simulink model "ROBOT_OK"  (R2021a)
settings: Solver=FixedStepAuto  StartTime=0.0  StopTime=inf  FixedStep=0.001  RelTol=1e-3
model workspace: external: MATLAB File E:\2024\TINH_TOAN_ROBOT_6_DOF\ROBOT_OK_DataFile.m (data not in the file)
values from neighbouring files (symbols this model uses):
  X = Toado(:,1)    [QuydaoK.m]
  Y = Toado(:,2)    [QuydaoK.m]
  Z = Toado(:,3)    [QuydaoK.m]
undefined symbols (not defined in the file or in its folder): smiData
libraries: sm_lib x38, nesl_utility x30, sharedutil x16, sharedtransform x12, dspmtrx3 x12, simulink_extras x8, pid_lib x6, simulink x3
(part 1 of 6)
settings Model: EnablePacing=on  Creator=NGAI-LAPTOP  LastModifiedBy=NGAI-LAPTOP

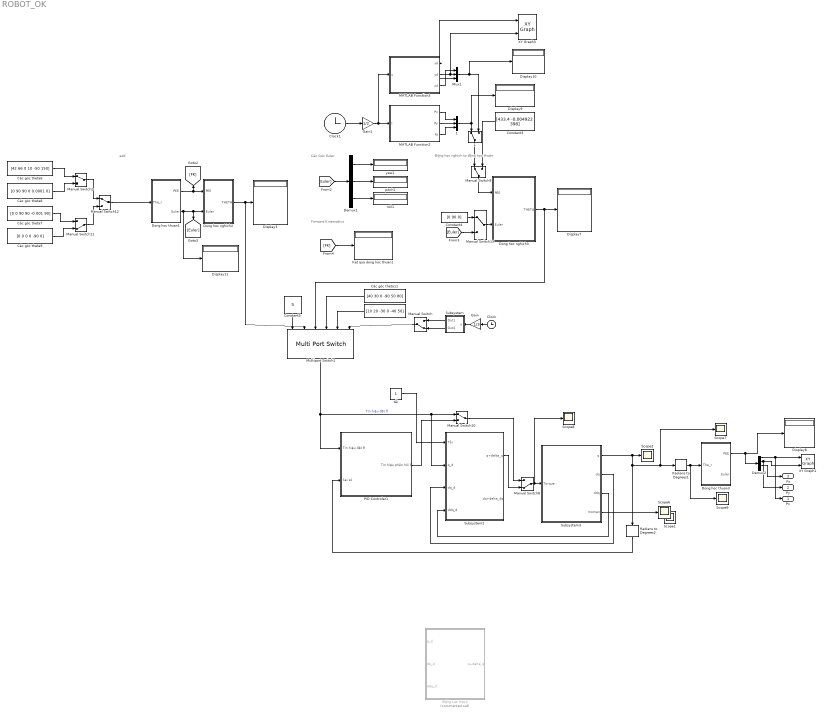
== system ROBOT_OK ==
  note: Động học nghịch to động học thuận
  note: Các Góc Euler
  note: add
  note: Forward Kinematics
  "   " : Constant  Value=[10 20 -30 0 -40 50]
  "   1" : Mux  Inputs=3
  " 1" : ManualSwitch
  Clock : Clock
  Clock1 : Clock
  Constant3 : Constant  Value=[433.4 -0.004922 398]
  Constant4 : Constant  Value=[0 90 0]
  Constant5 : Constant  Value=5
  Các góc theta11 : Constant  Value=[40 30 0 -90 50 80]
  Các góc theta6 : Constant  Value=[42 66 0 10 -50 150]
  Các góc theta7 : Constant  Value=[0 0 90 90 -0.001 90]
  Các góc theta8 : Constant  Value=[0 90 90 0 0.0001 0]
  Các góc theta9 : Constant  Value=[0 0 0 0 -90 0]
  Demux1 : Demux  Outputs=3
  Demux2 : Demux
  Display{3,7..11} (6 alike) : Display
  Dong hoc nghich2 : Subsystem
  Dong hoc nghich3 : Subsystem
  Dong hoc thuan1 : Subsystem
  Dong hoc thuan3 : Subsystem
  Gain : Gain  Gain=1/3
  Gain1 : Gain  Gain=1/2
  Ket qua dong hoc thuan1 : Display
  MATLAB Function2 : MATLAB Function  TreatAsAtomicUnit=on
  MATLAB Function3 : MATLAB Function  TreatAsAtomicUnit=on
  Manual Switch : ManualSwitch  CurrentSetting=0
  Manual Switch{2,9..10,12..13} (5 alike) : ManualSwitch
  Manual Switch11 : ManualSwitch  CurrentSetting=0
  Manual Switch8 : ManualSwitch  CurrentSetting=0
  Multiport Switch1 : MultiPortSwitch  Inputs=5
  Mux1 : Mux  Inputs=3
  PID Controler1 : Subsystem
  Radians to Degrees1 : simulink_extras/Transformations/Radians to Degrees
  Radians to Degrees2 : simulink_extras/Transformations/Radians to Degrees
  Scope{1..2,6..9} (6 alike) : Scope
  Subsystem : Subsystem
  Subsystem2 : Subsystem
  Subsystem3 : Subsystem
  XY Graph1 : simulink/Sinks/XY Graph  xmin=-1000  xmax=1000  ymin=-1000  ymax=1000  st=-1
  XY Graph3 : simulink/Sinks/XY Graph  xmin=-1  xmax=1  ymin=-1  ymax=1  st=-1
  pitch1 : Display
  roll1 : Display
  tải : Constant
  yaw1 : Display
  Động Lực Học2 : Subsystem  Commented=on
  Px : Outport
  Py : Outport  Port=2
  Pz : Outport  Port=3
  wires:
  MATLAB Function3/1(xd) -> Mux1/3, XY Graph3/1
  Các góc theta7/1 -> Manual Switch11/1
  Demux2/3 -> Pz/1
  Demux2/1 -> XY Graph1/1, Px/1
  Manual Switch9/1 -> Dong hoc nghich3/1(PEE)
  Manual Switch8/1 -> Subsystem3/1(Torque), Scope8/1
  Demux1/1 -> yaw1/1
  Manual Switch2/1 -> Manual Switch12/1
  Manual Switch13/1 -> Dong hoc nghich3/2(Euler)
  Subsystem3/4(momen) -> Scope6/1
  Dong hoc thuan3/1(PEE) -> Demux2/1, Display8/1
  [Euler] -> Demux1/1
  Các góc theta6/1 -> Manual Switch2/1
  PID Controler1/1(Tín hiệu phản hồi θ) -> Manual Switch10/2
  Multiport Switch1/1 -> Subsystem2/2(q_d), Manual Switch10/1, PID Controler1/1(Tín hiệu đặt θ)  "Tín hiệu đặt θ"
  Constant4/1 -> Manual Switch13/1
  Constant5/1 -> Multiport Switch1/1
  Radians to Degrees2/1 -> PID Controler1/2(Sai số)
  [FK] -> Ket qua dong hoc thuan1/1
  Manual Switch11/1 -> Manual Switch12/2
  Manual Switch10/1 -> Manual Switch8/1
  Các góc theta11/1 -> Multiport Switch1/4
  Các góc theta9/1 -> Manual Switch11/2
  "   "/1 -> Multiport Switch1/5
  Subsystem2/1(q+delta_q) -> Manual Switch8/2
  [Euler] -> Manual Switch13/2
  " 1"/1 -> Manual Switch9/1
  Subsystem3/2(dq) -> Subsystem2/3(dq_d)
  MATLAB Function3/3(zd) -> Mux1/1
  MATLAB Function3/2(yd) -> Mux1/2, XY Graph3/2
  MATLAB Function2/2(Py) -> "   1"/2
  Subsystem3/3(ddq) -> Subsystem2/4(ddq_d)
  Dong hoc thuan1/1(PEE) -> Dong hoc nghich2/1(PEE), [FK]
  "   1"/1 -> Display9/1, " 1"/1
  Mux1/1 -> " 1"/2, Display10/1
  MATLAB Function2/1(Px) -> "   1"/1
  Demux1/2 -> pitch1/1
  Demux1/3 -> roll1/1
  Gain1/1 -> MATLAB Function3/1(u), MATLAB Function2/1(t)
  MATLAB Function2/3(Pz) -> "   1"/3
  Constant3/1 -> Manual Switch9/2
  Subsystem3/1(q) -> Scope2/1, Radians to Degrees2/1, Radians to Degrees1/1, Scope7/1
  Manual Switch12/1 -> Dong hoc thuan1/1(The_r)
  Dong hoc thuan1/2(Euler) -> Dong hoc nghich2/2(Euler), [Euler], Display11/1
  Các góc theta8/1 -> Manual Switch2/2
  Dong hoc nghich3/1(THETA) -> Multiport Switch1/3, Display7/1
  Dong hoc nghich2/1(THETA) -> Multiport Switch1/2, Display3/1
  Clock1/1 -> Gain1/1
  Radians to Degrees1/1 -> Dong hoc thuan3/1(The_r), Scope9/1
  Demux2/2 -> XY Graph1/2, Py/1
  Subsystem/1(Out1) -> Manual Switch/1
  Subsystem/2(Out2) -> Manual Switch/2
  Manual Switch/1 -> Multiport Switch1/6
  Gain/1 -> Subsystem/1(u)
  Clock/1 -> Gain/1
  tải/1 -> Subsystem2/1(Tải)

== system ROBOT_OK/Dong hoc nghich2 ==
  PEE : Inport
  Euler : Inport  Port=2
  DONG HOC NGHICH : MATLAB Function  TreatAsAtomicUnit=on
  Demux : Demux  Outputs=3
  Display : Display
  Display1 : Display
  Mux : Mux  Inputs=6
  THETA : Outport
  wires:
  Demux/3 -> DONG HOC NGHICH/4(roll)
  Demux/1 -> DONG HOC NGHICH/2(yaw)
  Demux/2 -> DONG HOC NGHICH/3(pitch)
  DONG HOC NGHICH/3(the3) -> Mux/3
  DONG HOC NGHICH/4(the4) -> Mux/4
  DONG HOC NGHICH/2(the2) -> Mux/2
  DONG HOC NGHICH/6(the6) -> Mux/6
  DONG HOC NGHICH/5(the5) -> Mux/5
  PEE/1 -> Display/1, DONG HOC NGHICH/1(P_EE)
  Euler/1 -> Display1/1, Demux/1
  DONG HOC NGHICH/1(the1) -> Mux/1
  Mux/1 -> THETA/1

== system ROBOT_OK/Dong hoc nghich3 ==
  PEE : Inport
  Euler : Inport  Port=2
  DONG HOC NGHICH : MATLAB Function  TreatAsAtomicUnit=on
  Demux : Demux  Outputs=3
  Display : Display
  Display1 : Display
  Mux : Mux  Inputs=6
  THETA : Outport
  wires:
  Demux/3 -> DONG HOC NGHICH/4(roll)
  Demux/1 -> DONG HOC NGHICH/2(yaw)
  Demux/2 -> DONG HOC NGHICH/3(pitch)
  DONG HOC NGHICH/3(the3) -> Mux/3
  DONG HOC NGHICH/4(the4) -> Mux/4
  DONG HOC NGHICH/2(the2) -> Mux/2
  DONG HOC NGHICH/6(the6) -> Mux/6
  DONG HOC NGHICH/5(the5) -> Mux/5
  PEE/1 -> Display/1, DONG HOC NGHICH/1(P_EE)
  Euler/1 -> Display1/1, Demux/1
  DONG HOC NGHICH/1(the1) -> Mux/1
  Mux/1 -> THETA/1

== system ROBOT_OK/Dong hoc thuan1 ==
  The_r : Inport
  DONG HOC THUAN : MATLAB Function  TreatAsAtomicUnit=on
  Demux : Demux  Outputs=6
  Mux : Mux  Inputs=3
  PEE : Outport  VectorParamsAs1DForOutWhenUnconnected=off
  Euler : Outport  Port=2  VectorParamsAs1DForOutWhenUnconnected=off
  wires:
  Demux/5 -> DONG HOC THUAN/5(the5)
  Demux/1 -> DONG HOC THUAN/1(the1)
  Demux/4 -> DONG HOC THUAN/4(the4)
  DONG HOC THUAN/4(roll) -> Mux/3
  Demux/2 -> DONG HOC THUAN/2(the2)
  Demux/3 -> DONG HOC THUAN/3(the3)
  Demux/6 -> DONG HOC THUAN/6(the6)
  The_r/1 -> Demux/1
  DONG HOC THUAN/2(yaw) -> Mux/1
  DONG HOC THUAN/3(pitch) -> Mux/2
  Mux/1 -> Euler/1
  DONG HOC THUAN/1(P_EE) -> PEE/1

== system ROBOT_OK/Dong hoc thuan3 ==
  The_r : Inport
  DONG HOC THUAN : MATLAB Function  TreatAsAtomicUnit=on
  Demux : Demux  Outputs=6
  Mux : Mux  Inputs=3
  PEE : Outport  VectorParamsAs1DForOutWhenUnconnected=off
  Euler : Outport  Port=2  VectorParamsAs1DForOutWhenUnconnected=off
  wires:
  Demux/5 -> DONG HOC THUAN/5(the5)
  Demux/1 -> DONG HOC THUAN/1(the1)
  Demux/4 -> DONG HOC THUAN/4(the4)
  DONG HOC THUAN/4(roll) -> Mux/3
  Demux/2 -> DONG HOC THUAN/2(the2)
  Demux/3 -> DONG HOC THUAN/3(the3)
  Demux/6 -> DONG HOC THUAN/6(the6)
  The_r/1 -> Demux/1
  DONG HOC THUAN/2(yaw) -> Mux/1
  DONG HOC THUAN/3(pitch) -> Mux/2
  Mux/1 -> Euler/1
  DONG HOC THUAN/1(P_EE) -> PEE/1

== system ROBOT_OK/PID Controler1 ==
  Tín hiệu đặt θ : Inport
  Sai số : Inport  Port=2
  Demux1 : Demux  Outputs=6
  Mux : Mux  Inputs=6
  PID Controller1 : pid_lib/PID Controller  Controller=PID  Form=Parallel  TimeDomain=Continuous-time  UseExternalTs=off  SampleTime=-1  IntegratorMethod=Forward Euler  FilterMethod=Forward Euler  ControllerParametersSource=internal  P=0  I=9.99999999999999  D=0  UseFilter=on  N=100  TunerSelectOption=Transfer Function Based (PID Tuner App)  InitialConditionSource=internal  InitialConditionForIntegrator=0  InitialConditionForFilter=0  DifferentiatorICPrevScaledInput=0  ExternalReset=none  TrackingMode=off  Kt=1  LimitOutput=off  SatLimitsSource=internal  UpperSaturationLimit=inf  LowerSaturationLimit=-inf  LinearizeAsGain=on  AntiWindupMode=none  Kb=1  POutMin=[]  POutMax=[]  IOutMin=[]  IOutMax=[]  DOutMin=[]  DOutMax=[]  NOutMin=[]  NOutMax=[]  SumOutMin=[]  SumOutMax=[]  SaturationOutMin=[]  SaturationOutMax=[]  PParamMin=[]  PParamMax=[]  IParamMin=[]  IParamMax=[]  DParamMin=[]  DParamMax=[]  NParamMin=[]  NParamMax=[]  KbParamMin=[]  KbParamMax=[]  KtParamMin=[]  KtParamMax=[]  KbOutMin=[]  KbOutMax=[]  KtOutMin=[]  KtOutMax=[]  IntegratorOutMin=[]  IntegratorOutMax=[]  FilterOutMin=[]  FilterOutMax=[]  SumI1OutMin=[]  SumI1OutMax=[]  SumI2OutMin=[]  SumI2OutMax=[]  SumI3OutMin=[]  SumI3OutMax=[]  SumI4OutMin=[]  SumI4OutMax=[]  SumDOutMin=[]  SumDOutMax=[]  DifferentiatorOutMin=[]  DifferentiatorOutMax=[]  FilterDiffOutCoefMin=[]  FilterDiffOutCoefMax=[]  ReciprocalOutMin=[]  ReciprocalOutMax=[]  SumDenOutMin=[]  SumDenOutMax=[]  SumNumOutMin=[]  SumNumOutMax=[]  DivideOutMin=[]  DivideOutMax=[]  UdiffTsProdOutMin=[]  UdiffTsProdOutMax=[]  NTsProdOutMin=[]  NTsProdOutMax=[]  UintegralTsProdOutMin=[]  UintegralTsProdOutMax=[]  UngainTsProdOutMin=[]  UngainTsProdOutMax=[]  IntegratorContinuousStateAttributes=''  IntegratorStateMustResolveToSignalObject=off  IntegratorRTWStateStorageClass=Auto  FilterContinuousStateAttributes=''  FilterStateMustResolveToSignalObject=off  FilterRTWStateStorageClass=Auto  ParallelPVariant=InternalParameters  IdealPVariant=Disabled  IVariant=InternalParameters  DVariant=InternalParameters  IntegratorVariant=Continuous  SatVariant=Disabled  AWVariant=Passthrough  PCopyVariant=Disabled  TRVariant=Disabled  FdbkBlocksVariant=Forward  IdealPFdbkVariant=Disabled  SatFdbkVariant=Disabled  DerivativeFilterVariant=ContFilter  NVariant=InternalParameters  NCopyVariant=Disabled  FilterICVariant=InternalICsFilter  IntegratorICVariant=InternalICs  ExternalResetVariant=Disabled  TRSumVariant=Passthrough  SumFdbkVariant=Disabled  SumVariant=Sum_PID  TsampFilterVariant=InternalTs  TsampNgainVariant=Passthrough  TsampIntegralVariant=Passthrough  ExternalSaturationOutDataTypeStr=Inherit: Same as second input
  PID Controller2 : pid_lib/PID Controller  Controller=PID  Form=Parallel  TimeDomain=Continuous-time  UseExternalTs=off  SampleTime=-1  IntegratorMethod=Forward Euler  FilterMethod=Forward Euler  ControllerParametersSource=internal  P=0  I=10  D=0  UseFilter=on  N=100  TunerSelectOption=Transfer Function Based (PID Tuner App)  InitialConditionSource=internal  InitialConditionForIntegrator=0  InitialConditionForFilter=0  DifferentiatorICPrevScaledInput=0  ExternalReset=none  TrackingMode=off  Kt=1  LimitOutput=off  SatLimitsSource=internal  UpperSaturationLimit=inf  LowerSaturationLimit=-inf  LinearizeAsGain=on  AntiWindupMode=none  Kb=1  POutMin=[]  POutMax=[]  IOutMin=[]  IOutMax=[]  DOutMin=[]  DOutMax=[]  NOutMin=[]  NOutMax=[]  SumOutMin=[]  SumOutMax=[]  SaturationOutMin=[]  SaturationOutMax=[]  PParamMin=[]  PParamMax=[]  IParamMin=[]  IParamMax=[]  DParamMin=[]  DParamMax=[]  NParamMin=[]  NParamMax=[]  KbParamMin=[]  KbParamMax=[]  KtParamMin=[]  KtParamMax=[]  KbOutMin=[]  KbOutMax=[]  KtOutMin=[]  KtOutMax=[]  IntegratorOutMin=[]  IntegratorOutMax=[]  FilterOutMin=[]  FilterOutMax=[]  SumI1OutMin=[]  SumI1OutMax=[]  SumI2OutMin=[]  SumI2OutMax=[]  SumI3OutMin=[]  SumI3OutMax=[]  SumI4OutMin=[]  SumI4OutMax=[]  SumDOutMin=[]  SumDOutMax=[]  DifferentiatorOutMin=[]  DifferentiatorOutMax=[]  FilterDiffOutCoefMin=[]  FilterDiffOutCoefMax=[]  ReciprocalOutMin=[]  ReciprocalOutMax=[]  SumDenOutMin=[]  SumDenOutMax=[]  SumNumOutMin=[]  SumNumOutMax=[]  DivideOutMin=[]  DivideOutMax=[]  UdiffTsProdOutMin=[]  UdiffTsProdOutMax=[]  NTsProdOutMin=[]  NTsProdOutMax=[]  UintegralTsProdOutMin=[]  UintegralTsProdOutMax=[]  UngainTsProdOutMin=[]  UngainTsProdOutMax=[]  IntegratorContinuousStateAttributes=''  IntegratorStateMustResolveToSignalObject=off  IntegratorRTWStateStorageClass=Auto  FilterContinuousStateAttributes=''  FilterStateMustResolveToSignalObject=off  FilterRTWStateStorageClass=Auto  ParallelPVariant=InternalParameters  IdealPVariant=Disabled  IVariant=InternalParameters  DVariant=InternalParameters  IntegratorVariant=Continuous  SatVariant=Disabled  AWVariant=Passthrough  PCopyVariant=Disabled  TRVariant=Disabled  FdbkBlocksVariant=Forward  IdealPFdbkVariant=Disabled  SatFdbkVariant=Disabled  DerivativeFilterVariant=ContFilter  NVariant=InternalParameters  NCopyVariant=Disabled  FilterICVariant=InternalICsFilter  IntegratorICVariant=InternalICs  ExternalResetVariant=Disabled  TRSumVariant=Passthrough  SumFdbkVariant=Disabled  SumVariant=Sum_PID  TsampFilterVariant=InternalTs  TsampNgainVariant=Passthrough  TsampIntegralVariant=Passthrough  ExternalSaturationOutDataTypeStr=Inherit: Same as second input
  PID Controller3 : pid_lib/PID Controller  Controller=PID  Form=Parallel  TimeDomain=Continuous-time  UseExternalTs=off  SampleTime=-1  IntegratorMethod=Forward Euler  FilterMethod=Forward Euler  ControllerParametersSource=internal  P=0  I=10  D=0  UseFilter=on  N=944.848611425355  TunerSelectOption=Transfer Function Based (PID Tuner App)  InitialConditionSource=internal  InitialConditionForIntegrator=0  InitialConditionForFilter=0  DifferentiatorICPrevScaledInput=0  ExternalReset=none  TrackingMode=off  Kt=1  LimitOutput=off  SatLimitsSource=internal  UpperSaturationLimit=inf  LowerSaturationLimit=-inf  LinearizeAsGain=on  AntiWindupMode=none  Kb=1  POutMin=[]  POutMax=[]  IOutMin=[]  IOutMax=[]  DOutMin=[]  DOutMax=[]  NOutMin=[]  NOutMax=[]  SumOutMin=[]  SumOutMax=[]  SaturationOutMin=[]  SaturationOutMax=[]  PParamMin=[]  PParamMax=[]  IParamMin=[]  IParamMax=[]  DParamMin=[]  DParamMax=[]  NParamMin=[]  NParamMax=[]  KbParamMin=[]  KbParamMax=[]  KtParamMin=[]  KtParamMax=[]  KbOutMin=[]  KbOutMax=[]  KtOutMin=[]  KtOutMax=[]  IntegratorOutMin=[]  IntegratorOutMax=[]  FilterOutMin=[]  FilterOutMax=[]  SumI1OutMin=[]  SumI1OutMax=[]  SumI2OutMin=[]  SumI2OutMax=[]  SumI3OutMin=[]  SumI3OutMax=[]  SumI4OutMin=[]  SumI4OutMax=[]  SumDOutMin=[]  SumDOutMax=[]  DifferentiatorOutMin=[]  DifferentiatorOutMax=[]  FilterDiffOutCoefMin=[]  FilterDiffOutCoefMax=[]  ReciprocalOutMin=[]  ReciprocalOutMax=[]  SumDenOutMin=[]  SumDenOutMax=[]  SumNumOutMin=[]  SumNumOutMax=[]  DivideOutMin=[]  DivideOutMax=[]  UdiffTsProdOutMin=[]  UdiffTsProdOutMax=[]  NTsProdOutMin=[]  NTsProdOutMax=[]  UintegralTsProdOutMin=[]  UintegralTsProdOutMax=[]  UngainTsProdOutMin=[]  UngainTsProdOutMax=[]  IntegratorContinuousStateAttributes=''  IntegratorStateMustResolveToSignalObject=off  IntegratorRTWStateStorageClass=Auto  FilterContinuousStateAttributes=''  FilterStateMustResolveToSignalObject=off  FilterRTWStateStorageClass=Auto  ParallelPVariant=InternalParameters  IdealPVariant=Disabled  IVariant=InternalParameters  DVariant=InternalParameters  IntegratorVariant=Continuous  SatVariant=Disabled  AWVariant=Passthrough  PCopyVariant=Disabled  TRVariant=Disabled  FdbkBlocksVariant=Forward  IdealPFdbkVariant=Disabled  SatFdbkVariant=Disabled  DerivativeFilterVariant=ContFilter  NVariant=InternalParameters  NCopyVariant=Disabled  FilterICVariant=InternalICsFilter  IntegratorICVariant=InternalICs  ExternalResetVariant=Disabled  TRSumVariant=Passthrough  SumFdbkVariant=Disabled  SumVariant=Sum_PID  TsampFilterVariant=InternalTs  TsampNgainVariant=Passthrough  TsampIntegralVariant=Passthrough  ExternalSaturationOutDataTypeStr=Inherit: Same as second input
  PID Controller4 : pid_lib/PID Controller  Controller=PID  Form=Parallel  TimeDomain=Continuous-time  UseExternalTs=off  SampleTime=-1  IntegratorMethod=Forward Euler  FilterMethod=Forward Euler  ControllerParametersSource=internal  P=0  I=10  D=0  UseFilter=on  N=208.357752355368  TunerSelectOption=Transfer Function Based (PID Tuner App)  InitialConditionSource=internal  InitialConditionForIntegrator=0  InitialConditionForFilter=0  DifferentiatorICPrevScaledInput=0  ExternalReset=none  TrackingMode=off  Kt=1  LimitOutput=off  SatLimitsSource=internal  UpperSaturationLimit=inf  LowerSaturationLimit=-inf  LinearizeAsGain=on  AntiWindupMode=none  Kb=1  POutMin=[]  POutMax=[]  IOutMin=[]  IOutMax=[]  DOutMin=[]  DOutMax=[]  NOutMin=[]  NOutMax=[]  SumOutMin=[]  SumOutMax=[]  SaturationOutMin=[]  SaturationOutMax=[]  PParamMin=[]  PParamMax=[]  IParamMin=[]  IParamMax=[]  DParamMin=[]  DParamMax=[]  NParamMin=[]  NParamMax=[]  KbParamMin=[]  KbParamMax=[]  KtParamMin=[]  KtParamMax=[]  KbOutMin=[]  KbOutMax=[]  KtOutMin=[]  KtOutMax=[]  IntegratorOutMin=[]  IntegratorOutMax=[]  FilterOutMin=[]  FilterOutMax=[]  SumI1OutMin=[]  SumI1OutMax=[]  SumI2OutMin=[]  SumI2OutMax=[]  SumI3OutMin=[]  SumI3OutMax=[]  SumI4OutMin=[]  SumI4OutMax=[]  SumDOutMin=[]  SumDOutMax=[]  DifferentiatorOutMin=[]  DifferentiatorOutMax=[]  FilterDiffOutCoefMin=[]  FilterDiffOutCoefMax=[]  ReciprocalOutMin=[]  ReciprocalOutMax=[]  SumDenOutMin=[]  SumDenOutMax=[]  SumNumOutMin=[]  SumNumOutMax=[]  DivideOutMin=[]  DivideOutMax=[]  UdiffTsProdOutMin=[]  UdiffTsProdOutMax=[]  NTsProdOutMin=[]  NTsProdOutMax=[]  UintegralTsProdOutMin=[]  UintegralTsProdOutMax=[]  UngainTsProdOutMin=[]  UngainTsProdOutMax=[]  IntegratorContinuousStateAttributes=''  IntegratorStateMustResolveToSignalObject=off  IntegratorRTWStateStorageClass=Auto  FilterContinuousStateAttributes=''  FilterStateMustResolveToSignalObject=off  FilterRTWStateStorageClass=Auto  ParallelPVariant=InternalParameters  IdealPVariant=Disabled  IVariant=InternalParameters  DVariant=InternalParameters  IntegratorVariant=Continuous  SatVariant=Disabled  AWVariant=Passthrough  PCopyVariant=Disabled  TRVariant=Disabled  FdbkBlocksVariant=Forward  IdealPFdbkVariant=Disabled  SatFdbkVariant=Disabled  DerivativeFilterVariant=ContFilter  NVariant=InternalParameters  NCopyVariant=Disabled  FilterICVariant=InternalICsFilter  IntegratorICVariant=InternalICs  ExternalResetVariant=Disabled  TRSumVariant=Passthrough  SumFdbkVariant=Disabled  SumVariant=Sum_PID  TsampFilterVariant=InternalTs  TsampNgainVariant=Passthrough  TsampIntegralVariant=Passthrough  ExternalSaturationOutDataTypeStr=Inherit: Same as second input
  PID Controller5 : pid_lib/PID Controller  Controller=PID  Form=Parallel  TimeDomain=Continuous-time  UseExternalTs=off  SampleTime=-1  IntegratorMethod=Forward Euler  FilterMethod=Forward Euler  ControllerParametersSource=internal  P=0  I=10  D=0  UseFilter=on  N=100  TunerSelectOption=Transfer Function Based (PID Tuner App)  InitialConditionSource=internal  InitialConditionForIntegrator=0  InitialConditionForFilter=0  DifferentiatorICPrevScaledInput=0  ExternalReset=none  TrackingMode=off  Kt=1  LimitOutput=off  SatLimitsSource=internal  UpperSaturationLimit=inf  LowerSaturationLimit=-inf  LinearizeAsGain=on  AntiWindupMode=none  Kb=1  POutMin=[]  POutMax=[]  IOutMin=[]  IOutMax=[]  DOutMin=[]  DOutMax=[]  NOutMin=[]  NOutMax=[]  SumOutMin=[]  SumOutMax=[]  SaturationOutMin=[]  SaturationOutMax=[]  PParamMin=[]  PParamMax=[]  IParamMin=[]  IParamMax=[]  DParamMin=[]  DParamMax=[]  NParamMin=[]  NParamMax=[]  KbParamMin=[]  KbParamMax=[]  KtParamMin=[]  KtParamMax=[]  KbOutMin=[]  KbOutMax=[]  KtOutMin=[]  KtOutMax=[]  IntegratorOutMin=[]  IntegratorOutMax=[]  FilterOutMin=[]  FilterOutMax=[]  SumI1OutMin=[]  SumI1OutMax=[]  SumI2OutMin=[]  SumI2OutMax=[]  SumI3OutMin=[]  SumI3OutMax=[]  SumI4OutMin=[]  SumI4OutMax=[]  SumDOutMin=[]  SumDOutMax=[]  DifferentiatorOutMin=[]  DifferentiatorOutMax=[]  FilterDiffOutCoefMin=[]  FilterDiffOutCoefMax=[]  ReciprocalOutMin=[]  ReciprocalOutMax=[]  SumDenOutMin=[]  SumDenOutMax=[]  SumNumOutMin=[]  SumNumOutMax=[]  DivideOutMin=[]  DivideOutMax=[]  UdiffTsProdOutMin=[]  UdiffTsProdOutMax=[]  NTsProdOutMin=[]  NTsProdOutMax=[]  UintegralTsProdOutMin=[]  UintegralTsProdOutMax=[]  UngainTsProdOutMin=[]  UngainTsProdOutMax=[]  IntegratorContinuousStateAttributes=''  IntegratorStateMustResolveToSignalObject=off  IntegratorRTWStateStorageClass=Auto  FilterContinuousStateAttributes=''  FilterStateMustResolveToSignalObject=off  FilterRTWStateStorageClass=Auto  ParallelPVariant=InternalParameters  IdealPVariant=Disabled  IVariant=InternalParameters  DVariant=InternalParameters  IntegratorVariant=Continuous  SatVariant=Disabled  AWVariant=Passthrough  PCopyVariant=Disabled  TRVariant=Disabled  FdbkBlocksVariant=Forward  IdealPFdbkVariant=Disabled  SatFdbkVariant=Disabled  DerivativeFilterVariant=ContFilter  NVariant=InternalParameters  NCopyVariant=Disabled  FilterICVariant=InternalICsFilter  IntegratorICVariant=InternalICs  ExternalResetVariant=Disabled  TRSumVariant=Passthrough  SumFdbkVariant=Disabled  SumVariant=Sum_PID  TsampFilterVariant=InternalTs  TsampNgainVariant=Passthrough  TsampIntegralVariant=Passthrough  ExternalSaturationOutDataTypeStr=Inherit: Same as second input
  PID Controller6 : pid_lib/PID Controller  Controller=PID  Form=Parallel  TimeDomain=Continuous-time  UseExternalTs=off  SampleTime=-1  IntegratorMethod=Forward Euler  FilterMethod=Forward Euler  ControllerParametersSource=internal  P=0  I=10  D=0  UseFilter=on  N=100  TunerSelectOption=Transfer Function Based (PID Tuner App)  InitialConditionSource=internal  InitialConditionForIntegrator=0  InitialConditionForFilter=0  DifferentiatorICPrevScaledInput=0  ExternalReset=none  TrackingMode=off  Kt=1  LimitOutput=off  SatLimitsSource=internal  UpperSaturationLimit=inf  LowerSaturationLimit=-inf  LinearizeAsGain=on  AntiWindupMode=none  Kb=1  POutMin=[]  POutMax=[]  IOutMin=[]  IOutMax=[]  DOutMin=[]  DOutMax=[]  NOutMin=[]  NOutMax=[]  SumOutMin=[]  SumOutMax=[]  SaturationOutMin=[]  SaturationOutMax=[]  PParamMin=[]  PParamMax=[]  IParamMin=[]  IParamMax=[]  DParamMin=[]  DParamMax=[]  NParamMin=[]  NParamMax=[]  KbParamMin=[]  KbParamMax=[]  KtParamMin=[]  KtParamMax=[]  KbOutMin=[]  KbOutMax=[]  KtOutMin=[]  KtOutMax=[]  IntegratorOutMin=[]  IntegratorOutMax=[]  FilterOutMin=[]  FilterOutMax=[]  SumI1OutMin=[]  SumI1OutMax=[]  SumI2OutMin=[]  SumI2OutMax=[]  SumI3OutMin=[]  SumI3OutMax=[]  SumI4OutMin=[]  SumI4OutMax=[]  SumDOutMin=[]  SumDOutMax=[]  DifferentiatorOutMin=[]  DifferentiatorOutMax=[]  FilterDiffOutCoefMin=[]  FilterDiffOutCoefMax=[]  ReciprocalOutMin=[]  ReciprocalOutMax=[]  SumDenOutMin=[]  SumDenOutMax=[]  SumNumOutMin=[]  SumNumOutMax=[]  DivideOutMin=[]  DivideOutMax=[]  UdiffTsProdOutMin=[]  UdiffTsProdOutMax=[]  NTsProdOutMin=[]  NTsProdOutMax=[]  UintegralTsProdOutMin=[]  UintegralTsProdOutMax=[]  UngainTsProdOutMin=[]  UngainTsProdOutMax=[]  IntegratorContinuousStateAttributes=''  IntegratorStateMustResolveToSignalObject=off  IntegratorRTWStateStorageClass=Auto  FilterContinuousStateAttributes=''  FilterStateMustResolveToSignalObject=off  FilterRTWStateStorageClass=Auto  ParallelPVariant=InternalParameters  IdealPVariant=Disabled  IVariant=InternalParameters  DVariant=InternalParameters  IntegratorVariant=Continuous  SatVariant=Disabled  AWVariant=Passthrough  PCopyVariant=Disabled  TRVariant=Disabled  FdbkBlocksVariant=Forward  IdealPFdbkVariant=Disabled  SatFdbkVariant=Disabled  DerivativeFilterVariant=ContFilter  NVariant=InternalParameters  NCopyVariant=Disabled  FilterICVariant=InternalICsFilter  IntegratorICVariant=InternalICs  ExternalResetVariant=Disabled  TRSumVariant=Passthrough  SumFdbkVariant=Disabled  SumVariant=Sum_PID  TsampFilterVariant=InternalTs  TsampNgainVariant=Passthrough  TsampIntegralVariant=Passthrough  ExternalSaturationOutDataTypeStr=Inherit: Same as second input
  Sum : Sum  Inputs=|+-
  Tín hiệu phản hồi θ : Outport
  wires:
  PID Controller4/1 -> Mux/4
  PID Controller5/1 -> Mux/5
  Demux1/6 -> PID Controller6/1
  Demux1/3 -> PID Controller3/1
  PID Controller6/1 -> Mux/6
  Demux1/4 -> PID Controller4/1
  PID Controller3/1 -> Mux/3
  Sum/1 -> Demux1/1
  PID Controller1/1 -> Mux/1
  Demux1/5 -> PID Controller5/1
  PID Controller2/1 -> Mux/2
  Demux1/1 -> PID Controller1/1
  Demux1/2 -> PID Controller2/1
  Mux/1 -> Tín hiệu phản hồi θ/1  "Tín hiệu phản hồi θ"
  Tín hiệu đặt θ/1 -> Sum/1
  Sai số/1 -> Sum/2

== system ROBOT_OK/Subsystem ==
  u : Inport
  MATLAB Function1 : MATLAB Function  TreatAsAtomicUnit=on
  MATLAB Function4 : MATLAB Function  TreatAsAtomicUnit=on
  Mux : Mux  Inputs=6
  Mux2 : Mux  Inputs=6
  Out1 : Outport
  Out2 : Outport  Port=2
  wires:
  MATLAB Function1/6(y6) -> Mux2/6
  MATLAB Function4/5(y5) -> Mux/5
  MATLAB Function1/2(y2) -> Mux2/2
  MATLAB Function1/1(y1) -> Mux2/1
  u/1 -> MATLAB Function1/1(u), MATLAB Function4/1(u)
  MATLAB Function1/5(y5) -> Mux2/5
  MATLAB Function4/4(y4) -> Mux/4
  MATLAB Function1/4(y4) -> Mux2/4
  MATLAB Function1/3(y3) -> Mux2/3
  MATLAB Function4/2(y2) -> Mux/2
  MATLAB Function4/6(y6) -> Mux/6
  MATLAB Function4/3(y3) -> Mux/3
  MATLAB Function4/1(y1) -> Mux/1
  Mux2/1 -> Out1/1
  Mux/1 -> Out2/1

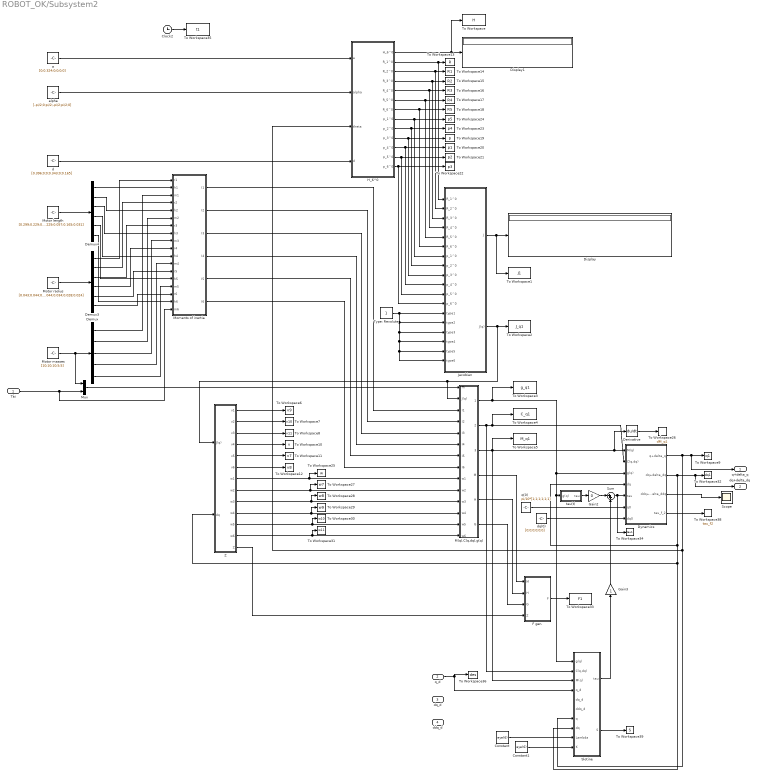
== system ROBOT_OK/Subsystem2 ==
  Tải : Inport
  q_d : Inport  Port=2
  dq_d : Inport  Port=3
  ddq_d : Inport  Port=4
  Clock2 : Clock
  Constant : Constant  Value=eye(6)
  Constant1 : Constant  Value=eye(6)
  Demux : Demux  Outputs=5
  Demux3 : Demux  Outputs=6
  Demux4 : Demux  Outputs=6
  Derivative : Derivative
  Display : Display
  Display1 : Display
  Dynamics : Subsystem
  F gen. : Subsystem
  Gain2 : Gain  Gain=0
  Gain3 : Gain
  H_6^0 : Subsystem
  Jacobian : Subsystem
  M(q),C(q,dq),g(q) : Subsystem
  Moments of inertia : Subsystem
  Motor length : Constant  Value=[0.299;0.229;0.229;0.057;0.165;0.031]
  Motor masses : Constant  Value=[10;10;10;5;5]
  Motor radius : Constant  Value=[0.043;0.044;0.044;0.034;0.028;0.024]
  Mux : Mux  Inputs=2
  Scope : Scope
  Slotine : Subsystem
  Sum : Sum  Inputs=|++
  To Workspace : ToWorkspace  VariableName=H  SampleTime=-1
  To Workspace1 : ToWorkspace  VariableName=J1  SampleTime=-1
  To Workspace10 : ToWorkspace  VariableName=v  SampleTime=-1
  To Workspace11 : ToWorkspace  VariableName=v7  SampleTime=-1
  To Workspace12 : ToWorkspace  VariableName=v8  SampleTime=-1
  To Workspace13 : ToWorkspace  VariableName=R  SampleTime=-1
  To Workspace14 : ToWorkspace  VariableName=R1  SampleTime=-1
  To Workspace15 : ToWorkspace  VariableName=R2  SampleTime=-1
  To Workspace16 : ToWorkspace  VariableName=R3  SampleTime=-1
  To Workspace17 : ToWorkspace  VariableName=R4  SampleTime=-1
  To Workspace18 : ToWorkspace  VariableName=R5  SampleTime=-1
  To Workspace19 : ToWorkspace  VariableName=p  SampleTime=-1
  To Workspace2 : ToWorkspace  VariableName=J_q1  SampleTime=-1
  To Workspace20 : ToWorkspace  VariableName=p1  SampleTime=-1
  To Workspace21 : ToWorkspace  VariableName=p2  SampleTime=-1
  To Workspace22 : ToWorkspace  VariableName=p3  SampleTime=-1
  To Workspace23 : ToWorkspace  VariableName=p4  SampleTime=-1
  To Workspace24 : ToWorkspace  VariableName=p5  SampleTime=-1
  To Workspace25 : ToWorkspace  VariableName=w  SampleTime=-1
  To Workspace26 : ToWorkspace  VariableName=dM_q1  SampleTime=-1
  To Workspace27 : ToWorkspace  VariableName=w7  SampleTime=-1
  To Workspace28 : ToWorkspace  VariableName=w8  SampleTime=-1
  To Workspace29 : ToWorkspace  VariableName=w9  SampleTime=-1
  To Workspace3 : ToWorkspace  VariableName=g_q1  SampleTime=-1
  To Workspace30 : ToWorkspace  VariableName=w10  SampleTime=-1
  To Workspace31 : ToWorkspace  VariableName=w11  SampleTime=-1
  To Workspace32 : ToWorkspace  VariableName=dq1  SampleTime=-1
  To Workspace33 : ToWorkspace  VariableName=F1  SampleTime=-1
  To Workspace34 : ToWorkspace  VariableName=tau1  SampleTime=-1
  To Workspace35 : ToWorkspace  VariableName=t1  SampleTime=-1
  To Workspace36 : ToWorkspace  VariableName=des  SampleTime=-1
  To Workspace38 : ToWorkspace  VariableName=tau_f2  SampleTime=-1
  To Workspace39 : ToWorkspace  VariableName=S  SampleTime=-1
  To Workspace4 : ToWorkspace  VariableName=C_q1  SampleTime=-1
  To Workspace5 : ToWorkspace  VariableName=M_q1  SampleTime=-1
  To Workspace6 : ToWorkspace  VariableName=v9  SampleTime=-1
  To Workspace7 : ToWorkspace  VariableName=v10  SampleTime=-1
  To Workspace8 : ToWorkspace  VariableName=v11  SampleTime=-1
  To Workspace9 : ToWorkspace  VariableName=q1  SampleTime=-1
  Type: Revolute : Constant
  Z : Subsystem
  a : Constant  Value=[0;0.324;0;0;0;0]
  alpha : Constant  Value=[-pi/2;0;pi/2;-pi/2;pi/2;0]
  d : Constant  Value=[0.396;0;0;0.343;0;0.165]
  dq(0) : Constant  Value=[0;0;0;0;0;0]
  q(0) : Constant  Value=pi/10*[1;1;1;1;1;1]
  tau(t) : Subsystem
  q+delta_q : Outport
  dq+delta_dq : Outport  Port=2
  wires:
  H_6^0/4(R_3^0) -> To Workspace15/1, Jacobian/3(R_3^0)
  Z/13(Z) -> F gen./4(Z)
  dq(0)/1 -> Dynamics/7(dq0)
  H_6^0/10(p_3^0) -> Jacobian/9(p_3^0), To Workspace19/1
  M(q),C(q,dq),g(q)/3(M(q)) -> Slotine/3(M(q)), To Workspace5/1, Derivative/1, Dynamics/1(M(q))
  Type: Revolute/1 -> Jacobian/14(type2), Jacobian/15(type3), Jacobian/18(type6), Jacobian/17(type5), Jacobian/16(type4), Jacobian/13(type1)
  Gain2/1 -> Sum/1
  Moments of inertia/6(I6) -> M(q),C(q,dq),g(q)/8(I6)
  tau(t)/1(tau) -> Gain2/1
  Moments of inertia/2(I2) -> M(q),C(q,dq),g(q)/4(I2)
  Constant1/1 -> Slotine/10(K)
  H_6^0/6(R_5^0) -> To Workspace17/1, Jacobian/5(R_5^0)
  Z/11(w5) -> To Workspace30/1, M(q),C(q,dq),g(q)/13(w5)
  H_6^0/1(H_6^0) -> To Workspace/1, Display1/1
  Tải/1 -> Mux/2, Moments of inertia/18(m6)
  H_6^0/5(R_4^0) -> To Workspace16/1, Jacobian/4(R_4^0)
  H_6^0/12(p_5^0) -> To Workspace21/1, Jacobian/11(p_5^0)
  q(0)/1 -> Dynamics/6(q0)
  Moments of inertia/1(I1) -> M(q),C(q,dq),g(q)/3(I1)
  Dynamics/1(q+delta_q) -> Slotine/7(q), H_6^0/3(theta), q+delta_q/1, To Workspace9/1
  Jacobian/2(J(q)) -> M(q),C(q,dq),g(q)/2(J(q)), Z/1(J(q)), To Workspace2/1
  Moments of inertia/4(I4) -> M(q),C(q,dq),g(q)/6(I4)
  Moments of inertia/5(I5) -> M(q),C(q,dq),g(q)/7(I5)
  Dynamics/4(tau_f_2) -> To Workspace38/1
  Z/8(w2) -> To Workspace27/1, M(q),C(q,dq),g(q)/10(w2)
  M(q),C(q,dq),g(q)/2(C(q,dq)) -> Slotine/2(C(q,dq)), To Workspace4/1, Dynamics/2(C(q,dq))
  Z/7(w1) -> To Workspace25/1, M(q),C(q,dq),g(q)/9(w1)
  Z/4(v4) -> To Workspace10/1
  Z/6(v6) -> To Workspace12/1
  Moments of inertia/3(I3) -> M(q),C(q,dq),g(q)/5(I3)
  H_6^0/11(p_4^0) -> To Workspace20/1, Jacobian/10(p_4^0)
  H_6^0/2(R_1^0) -> To Workspace13/1, Jacobian/1(R_1^0)
  Z/9(w3) -> To Workspace28/1, M(q),C(q,dq),g(q)/11(w3)
  M(q),C(q,dq),g(q)/1(g(q)) -> Dynamics/3(g(q)), tau(t)/1(g(q)), Slotine/1(g(q)), To Workspace3/1
  H_6^0/8(p_1^0) -> Jacobian/7(p_1^0), To Workspace24/1
  Z/2(v2) -> To Workspace7/1
  Mux/1 -> M(q),C(q,dq),g(q)/1(m)
  M(q),C(q,dq),g(q)/6(G) -> F gen./3(G)
  Demux3/2 -> Moments of inertia/4(r2)
  H_6^0/9(p_2^0) -> To Workspace23/1, Jacobian/8(p_2^0)
  Demux4/6 -> Moments of inertia/17(h6)
  Jacobian/1(J) -> To Workspace1/1, Display/1
  H_6^0/13(p_6^0) -> To Workspace22/1, Jacobian/12(p_6^0)
  Z/10(w4) -> To Workspace29/1, M(q),C(q,dq),g(q)/12(w4)
  Clock2/1 -> To Workspace35/1
  Demux4/4 -> Moments of inertia/11(h4)
  Demux/1 -> Moments of inertia/3(m1)
  Motor masses/1 -> Demux/1, Mux/1
  q_d/1 -> Slotine/4(q_d), To Workspace36/1
  Dynamics/2(dq+delta_dq) -> Z/2(dq), Slotine/8(dq), Dynamics/4(dq), dq+delta_dq/1, To Workspace32/1
  Demux3/4 -> Moments of inertia/10(r4)
  Z/1(v1) -> To Workspace6/1
  Sum/1 -> To Workspace34/1, Dynamics/5(tau)
  H_6^0/3(R_2^0) -> To Workspace14/1, Jacobian/2(R_2^0)
  Constant/1 -> Slotine/9(Lambda)
  Slotine/2(S) -> To Workspace39/1
  Demux3/5 -> Moments of inertia/13(r5)
  H_6^0/7(R_6^0) -> To Workspace18/1, Jacobian/6(R_6^0)
  M(q),C(q,dq),g(q)/4(M) -> F gen./1(M)
  Demux3/6 -> Moments of inertia/16(r6)
  Slotine/1(tau) -> Gain3/1
  F gen./1(F) -> To Workspace33/1
  Gain3/1 -> Sum/2
  a/1 -> H_6^0/1(a)
  Demux/3 -> Moments of inertia/9(m3)
  alpha/1 -> H_6^0/2(alpha)
  Derivative/1 -> To Workspace26/1
  Demux4/3 -> Moments of inertia/8(h3)
  Demux4/2 -> Moments of inertia/5(h2)
  d/1 -> H_6^0/4(d)
  Demux4/1 -> Moments of inertia/2(h1)
  Z/5(v5) -> To Workspace11/1
  Motor length/1 -> Demux4/1
  M(q),C(q,dq),g(q)/5(H) -> F gen./2(H)
  Motor radius/1 -> Demux3/1
  Demux4/5 -> Moments of inertia/14(h5)
  Z/12(w6) -> To Workspace31/1, M(q),C(q,dq),g(q)/14(w6)
  Demux/4 -> Moments of inertia/12(m4)
  Demux3/3 -> Moments of inertia/7(r3)
  Demux3/1 -> Moments of inertia/1(r1)
  Demux/5 -> Moments of inertia/15(m5)
  Demux/2 -> Moments of inertia/6(m2)
  Z/3(v3) -> To Workspace8/1
  Dynamics/3(ddq+delta_ddq) -> Scope/1
